simulink model "sltestTrafficLight"  (R2022a)
settings: Solver=FixedStepDiscrete  StartTime=0.0  StopTime=1000  FixedStep=0.1  RelTol=1e-3  EnableMultiTasking=on
undefined symbols (not defined in the file or in its folder): greenLightLocked, greenLightRequested, Hecate_Amp1, Hecate_Amp2, Hecate_delay, Hecate_Freq1, Hecate_Freq2
libraries: sltestTrafficLight_lib x5
settings Model: Creator=The MathWorks, Inc.  LastModifiedBy=fedformi_new
settings SolverCC: AlgebraicLoopSolver=TrustRegion
settings DataIOCC: SaveFormat=Array  ReturnWorkspaceOutputs=off
settings OptimizationCC: ExpressionDepthLimit=2147483647  InitFltsAndDblsToZero=on  EfficientMapNaN2IntZero=off  LifeSpan=inf
settings DebuggingCC: SaveWithParameterizedLinksMsg=none  UnderspecifiedInitializationDetection=Classic  MergeDetectMultiDrivingBlocksExec=none  SignalResolutionControl=TryResolveAllWithWarning  SolverPrmCheckMsg=warning  MultiTaskDSMMsg=warning  MultiTaskCondExecSysMsg=none  FcnCallInpInsideContextMsg=warning  UnconnectedInputMsg=warning  UnconnectedOutputMsg=warning  UnconnectedLineMsg=warning  StateNameClashWarn=warning  SFUnexpectedBacktrackingDiag=warning  SFNoUnconditionalDefaultTransitionDiag=warning  SFExecutionAtInitializationDiag=none  SFMachineParentedDataDiag=warning  ArithmeticOperatorsInVariantConditions=warning
settings HardwareCC: ProdBitPerPointer=32  ProdBitPerSizeT=32  ProdBitPerPtrDiffT=32  ProdLargestAtomicFloat=None  ProdIntDivRoundTo=Undefined  ProdEndianess=Unspecified  ProdWordSize=32  ProdHWDeviceType=32-bit Generic
settings ModelReferenceCC: PropagateSignalLabelsOutOfModel=off
settings SFSimCC: SimUseLocalCustomCode=off  SimParseCustomCode=off  CustomCodeUndefinedFunction=UseInterfaceOnly
settings RTWCC: RTWUseLocalCustomCode=off  DLArmComputeVersion=19.05
settings CodeAppCC: StateflowObjectComments=on
settings GRTTargetCC: TargetFcnLib=ansi_tfl_tmw.mat  TargetLangStandard=C89/C90 (ANSI)  CombineOutputUpdateFcns=off  GRTInterface=on
settings ConfigComp: CovMetricSettings=dw  CovSaveCumulativeToWorkspaceVar=on  CovSaveSingleToWorkspaceVar=on  CovExternalEMLEnable=off  CovSFcnEnable=off

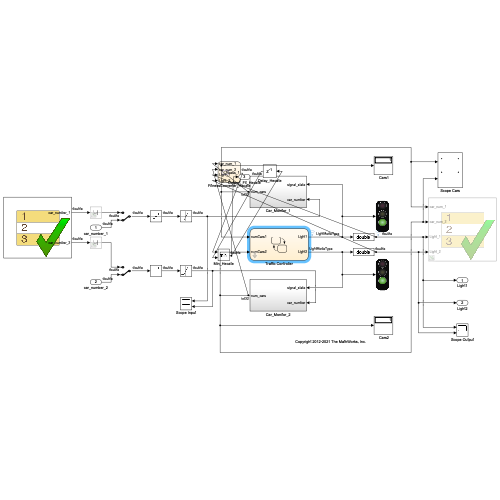
[thumbnail: Simulink's stored preview of the top-level diagram]
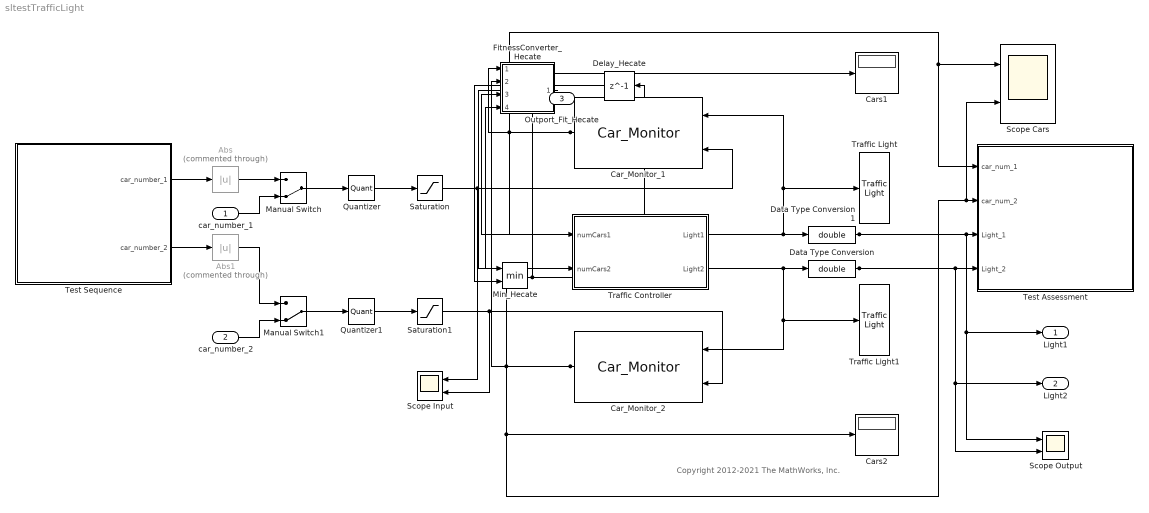
== system sltestTrafficLight ==
  note: Copyright 2012-2021 The MathWorks, Inc.
  car_number_1 : Inport
  car_number_2 : Inport  Port=2
  " Cars1" : Display
  " Cars2" : Display
  Abs : Abs  Commented=through  SaturateOnIntegerOverflow=off
  Abs1 : Abs  Commented=through  SaturateOnIntegerOverflow=off
  Car_Monitor_1 : sltestTrafficLight_lib/Car_Monitor  SystemSampleTime=-1  VariantActivationTime=update diagram  Latency=0  AutoFrameSizeCalculation=off
  Car_Monitor_2 : sltestTrafficLight_lib/Car_Monitor  SystemSampleTime=-1  VariantActivationTime=update diagram  Latency=0  AutoFrameSizeCalculation=off
  Data Type Conversion : DataTypeConversion  OutDataTypeStr=double  SaturateOnIntegerOverflow=off  RndMeth=Floor
  Data Type Conversion1 : DataTypeConversion  OutDataTypeStr=double  SaturateOnIntegerOverflow=off  RndMeth=Floor
  Delay_Hecate : Delay  DelayLength=1  InitialCondition=Inf
  FitnessConverter_Hecate : Stateflow chart  TreatAsAtomicUnit=on
  Manual Switch : ManualSwitch  CurrentSetting=0
  Manual Switch1 : ManualSwitch  CurrentSetting=0
  Min_Hecate : MinMax  Inputs=2
  Quantizer : Quantizer  QuantizationInterval=1
  Quantizer1 : Quantizer  QuantizationInterval=1
  Saturation : Saturate  UpperLimit=5  LowerLimit=0
  Saturation1 : Saturate  UpperLimit=5  LowerLimit=0
  Scope Cars : Scope  NumInputPorts=2
  Scope Input : Scope  NumInputPorts=2
  Scope Output : Scope  NumInputPorts=2
  Test Assessment : Test Sequence  TreatAsAtomicUnit=on
  Test Sequence : Test Sequence  TreatAsAtomicUnit=on
  Traffic Controller : Stateflow chart  TreatAsAtomicUnit=on  mask{REDDELAY=6, YELLOWDELAY=15, GREENDELAY=180, MINGREENDELAY=120, MAXREDDELAY=360}
  Traffic Light : sltestTrafficLight_lib/Traffic Light  mode=LightModeType.Green
  Traffic Light1 : sltestTrafficLight_lib/Traffic Light  mode=LightModeType.Green
  Light1 : Outport
  Light2 : Outport  Port=2
  Outport_Fit_Hecate : Outport  Port=3
  wires:
  Car_Monitor_2/1 -> Scope Cars/2, Test Assessment/2(car_num_2), " Cars2"/1, Traffic Controller/2(numCars2), FitnessConverter_Hecate/2(car_num_2)
  Car_Monitor_1/1 -> Test Assessment/1(car_num_1), Scope Cars/1, " Cars1"/1, Traffic Controller/1(numCars1), FitnessConverter_Hecate/1(car_num_1)
  Traffic Controller/2(Light2) -> Traffic Light1/1, Car_Monitor_2/1, Data Type Conversion/1
  Traffic Controller/1(Light1) -> Traffic Light/1, Car_Monitor_1/1, Data Type Conversion1/1
  car_number_1/1 -> Manual Switch/2
  Test Sequence/1(car_number_1) -> Abs/1
  car_number_2/1 -> Manual Switch1/2
  Test Sequence/2(car_number_2) -> Abs1/1
  Manual Switch1/1 -> Quantizer1/1
  Manual Switch/1 -> Quantizer/1
  Quantizer/1 -> Saturation/1
  Quantizer1/1 -> Saturation1/1
  Data Type Conversion/1 -> Test Assessment/4(Light_2), Scope Output/2, Light2/1, FitnessConverter_Hecate/4(Light_2)
  Data Type Conversion1/1 -> Scope Output/1, Light1/1, Test Assessment/3(Light_1), FitnessConverter_Hecate/3(Light_1)
  Saturation/1 -> Car_Monitor_1/2, Scope Input/1
  Saturation1/1 -> Scope Input/2, Car_Monitor_2/2
  Abs/1 -> Manual Switch/1
  Abs1/1 -> Manual Switch1/1
  FitnessConverter_Hecate/1(fitness_1) -> Min_Hecate/1
  Min_Hecate/1 -> Delay_Hecate/1, Outport_Fit_Hecate/1
  Delay_Hecate/1 -> Min_Hecate/2

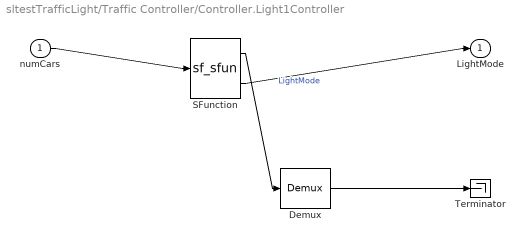
== system sltestTrafficLight/Traffic Controller/Controller.Light1Controller ==
  numCars : Inport
  " Demux " : Demux  Outputs=1
  " SFunction " : S-Function  Tag=Stateflow S-Function 5  FunctionName=sf_sfun  Parameters=GREENDELAY,MAXREDDELAY,MINGREENDELAY,REDDELAY,YELLOWDELAY  PortCounts=[1 2]  SFunctionDeploymentMode=off  EnableBusSupport=off
  " Terminator " : Terminator
  LightMode : Outport  VectorParamsAs1DForOutWhenUnconnected=off
  wires:
  numCars/1 -> " SFunction "/1
  " SFunction "/2 -> LightMode/1  "LightMode"
  " Demux "/1 -> " Terminator "/1
  " SFunction "/1 -> " Demux "/1

== stateflow chart sltestTrafficLight/Traffic Controller ==
  state Controller
    state Light1Controller [parallel]
      settings: executionOrder=1
    state Light2Controller [parallel]
      settings: executionOrder=2
  data: numCars1 input; numCars2 input; GREENDELAY parameter; MAXREDDELAY parameter; REDDELAY parameter; YELLOWDELAY parameter; MINGREENDELAY parameter; Light1 output Enum: LightModeType; greenLightLocked local boolean; greenLightRequested local boolean; Light2 output Enum: LightModeType

== stateflow chart sltestTrafficLight/Test Assessment ==
  state Req_1
    state step_1
      verify(car_num_1 >=0 && car_num_2 >= 0)
    (default) -> Req_1.step_1
  state Req_2
    state step_1
      verify(Light_1 >= 1.6 || Light_2 >= 1.7)
      settings: description=|
          | Traffic light conversion double - LightModeType
          |    0 = Green
          |    1 = Yellow
          |    2 = Red
    (default) -> Req_2.step_1
  state Req_3
    state step_1
    state step_2
    state step_3
      verify(true)
    state step_4
      verify(false)
    (default) -> Req_3.step_1
    (junction 96) -> Req_3.step_1
    (junction 98) -> (junction 96)
    Req_3.step_1 -> step_2 : [
        | Light_1 == LightModeType.Yellow
        | ]
    step_2 -> step_3 [order 1] : [
        | Light_1 == LightModeType.Red
        | ]
    step_2 -> (junction 107) [order 2] : [
        | et >= YellowDelayWithTol
        | ]
    step_3 -> (junction 98)
    (junction 102) -> (junction 98)
    step_4 -> (junction 102)
    (junction 105) -> step_4
    (junction 107) -> (junction 105)
  (default) -> Req_1 [order 1] : [Active_Scenario_Index == 1]
  (default) -> Req_2 [order 2] : [Active_Scenario_Index == 2]
  (default) -> Req_3 [order 3] : {assert(Active_Scenario_Index == 3,'The value of Scenario Parameter ''Active_Scenario_Index'' is not valid. Use the index of the scenario to specify it.')}
  data: Active_Scenario_Index parameter =2; car_num_1 input; car_num_2 input; Light_1 input; Light_2 input; YellowDelayWithTol constant double =15.5

== stateflow chart sltestTrafficLight/FitnessConverter_Hecate ==
  state step_1
    fitness_1 = max([Light_1-(1.6);Light_2-(1.7);]);
  (default) -> step_1
  data: car_num_1 input; car_num_2 input; Light_1 input; Light_2 input; fitness_1 output

== stateflow chart sltestTrafficLight/Test Sequence ==
  state step_1
    car_number_1 = Hecate_Amp1*sin(2*pi*Hecate_Freq1*t);
    car_number_2 = Hecate_Amp2*sin(2*pi*Hecate_Freq2*(t+Hecate_delay));
    settings: description=car_number always between 0 and 5 (included)
    state step_1_1
    (default) -> step_1_1
  (default) -> step_1
  data: car_number_1 output; car_number_2 output; Hecate_Amp1 parameter; Hecate_Amp2 parameter; Hecate_Freq1 parameter; Hecate_Freq2 parameter; Hecate_delay parameter

== stateflow chart sltestTrafficLight/Traffic Controller/Controller.Light1Controller ==
  state Red
    state DelayState
    state WaitForInput
    state WaitUntilSafeToChange
      du: greenLightRequested = true;
    (default) -> DelayState
    DelayState -> WaitForInput : [after(REDDELAY, sec)]
    WaitForInput -> WaitUntilSafeToChange [order 1] : [numCars > 0]
    WaitForInput -> WaitUntilSafeToChange [order 2] : [after(MAXREDDELAY,sec)]
  state Yellow
    ex:
    greenLightLocked = false;
  state Green
    en: greenLightLocked = true;
    greenLightRequested = false;
  (default) -> Red
  WaitUntilSafeToChange -> Green [order 1] : [after(130,sec)]
  WaitUntilSafeToChange -> (junction 92) [order 2] : [~greenLightLocked ...
      | && after(REDDELAY-5,sec)]
  Yellow -> Red : [after(YELLOWDELAY,sec)]
  Green -> Yellow [order 2] : [after(MINGREENDELAY, sec)...
      | && greenLightRequested]
  Green -> Yellow [order 1] : [after(GREENDELAY,sec)]
  (junction 92) -> Green
  data: numCars input; GREENDELAY parameter; MAXREDDELAY parameter; REDDELAY parameter; YELLOWDELAY parameter; MINGREENDELAY parameter; greenLightLocked data_store_memory; greenLightRequested data_store_memory; LightMode output Enum: LightModeType
